simulink model "D3exam"  (R2017b)
settings: Solver=VariableStepAuto  StartTime=0.0  StopTime=10.0  RelTol=1e-3
libraries: shared3dof x1
settings Model: Creator=ken  LastModifiedBy=ken

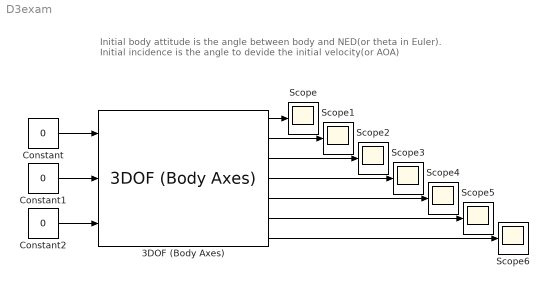
== system D3exam ==
  note: Initial body attitude is the angle between body and NED(or theta in Euler).
      | Initial incidence is the angle to devide the initial velocity(or AOA)
  3DOF (Body Axes) : shared3dof/3DOF (Body Axes)  units=Metric (MKS)  mtype=Fixed  v_ini=100  theta_ini=0  alpha_ini=-10*pi/180  q_ini=0  pos_ini=[0 0]  mass=1.0  mass_e=0.5  mass_f=3.0  Iyy=1.0  Iyy_e=0.5  Iyy_f=3.0  g_in=Internal  g=0  vre_flag=on  abi_flag=on
      settings: SourceProductName=Aerospace Blockset  SourceProductBaseCode=AE
  Constant : Constant  Value=0
  Constant1 : Constant  Value=0
  Constant2 : Constant  Value=0
  Scope{,1..6} (7 alike) : Scope
  wires:
  3DOF (Body Axes)/2 -> Scope1/1
  3DOF (Body Axes)/4 -> Scope3/1
  3DOF (Body Axes)/3 -> Scope2/1
  Constant2/1 -> 3DOF (Body Axes)/3
  3DOF (Body Axes)/5 -> Scope4/1
  Constant/1 -> 3DOF (Body Axes)/1
  3DOF (Body Axes)/6 -> Scope5/1
  3DOF (Body Axes)/7 -> Scope6/1
  Constant1/1 -> 3DOF (Body Axes)/2
  3DOF (Body Axes)/1 -> Scope/1
